simulink model "lqr_model"  (R2021a)
settings: Solver=VariableStepAuto  StartTime=0.0  StopTime=20  FixedStep=0.01  RelTol=1e-3
values from neighbouring files (symbols this model uses):
  FF_L = op.inputs(1).u    [trim_boat.m]
  initial_P = op.states(7).x    [trim_boat.m]
  initial_Q = op.states(3).x    [trim_boat.m]
  initial_R = op.states(8).x    [trim_boat.m]
  initial_uspeed = op.states(1).x    [trim_boat.m]
  initial_vspeed = op.states(6).x    [trim_boat.m]
  initial_wspeed = op.states(2).x    [trim_boat.m]
  initial_Z = op.states(5).x    [trim_boat.m]
  rear_alfas = op.inputs(3).u    [trim_boat.m]
  T = op.inputs(4).u    [trim_boat.m]
undefined symbols (not defined in the file or in its folder): ap2, ar2, ay2, bp2, br2, by2, Eff, K
libraries: simulink x4, pid_lib x1, dsparch4 x1
(part 2 of 2)

== matlab function lqr_model/SensorNoise/MATLAB Function ==
  data: u input; vz output; w input; Pitch input
function vz = fcn(u,w,Pitch)

Roll = 0;
Yaw = 0;

%Inertial to body frame matrix
R = [cosd(Pitch)*cosd(Yaw) cosd(Pitch)*sind(Yaw) -sind(Pitch);
    sind(Roll)*sind(Pitch)*cosd(Yaw)-cosd(Roll)*sind(Yaw) sind(Roll)*sind(Pitch)*sind(Yaw)+cosd(Roll)*cosd(Yaw) sind(Roll)*cosd(Pitch);
    cosd(Roll)*sind(Pitch)*cosd(Yaw)+sind(Roll)*sind(Yaw) cosd(Roll)*sind(Pitch)*sind(Yaw)-sind(Roll)*cosd(Yaw) cosd(Roll)*cosd(Pitch)];

VI_dot = R*[u;0;w];

vz = VI_dot(3);
